simulink model "Fact"  (R2021a)
settings: Solver=VariableStepAuto  StartTime=0.0  StopTime=10.0  RelTol=1e-3
settings Model: Creator=pc  LastModifiedBy=pc

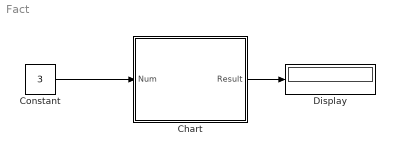
== system Fact ==
  Chart : Stateflow chart  TreatAsAtomicUnit=on
  Constant : Constant  Value=3
  Display : Display
  wires:
  Constant/1 -> Chart/1(Num)
  Chart/1(Result) -> Display/1

== stateflow chart Fact/Chart ==
  (default) -> (junction 10) : % Fact
      | {Fact=uint16(1);
      | Loop=Num;
      | }
  (junction 10) -> (junction 12) : {index=1;}
  (junction 12) -> (junction 11) [order 1] : [index<Num]
  (junction 11) -> (junction 13) : {Fact=Fact*Loop;
      | Loop=Loop-1;}
  (junction 14) -> (junction 12)
  (junction 12) -> (junction 15) [order 2] : {Result=Fact;}
  (junction 13) -> (junction 14) : {index=index+1;}
  data: Num input; Result output; Fact local; index local; Loop local
